simulink model "sample"  (R2018b)
settings: Solver=FixedStepDiscrete  StartTime=0.0  StopTime=10.0  RelTol=1e-3
settings Model: Creator=a_miyazaki  LastModifiedBy=a_miyazaki

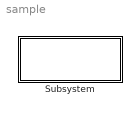
== system sample ==
  Subsystem : Subsystem

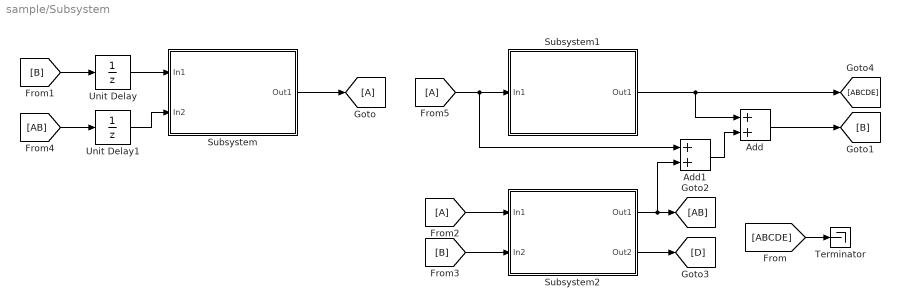
== system sample/Subsystem ==
  Add : Sum
  Add1 : Sum
  Subsystem : Subsystem
  Subsystem1 : Subsystem
  Subsystem2 : Subsystem
  Terminator : Terminator
  Unit Delay : UnitDelay  SampleTime=-1
  Unit Delay1 : UnitDelay  SampleTime=-1
  wires:
  Subsystem2/2(Out2) -> [D]
  [AB] -> Unit Delay1/1
  Add/1 -> [B]
  Unit Delay1/1 -> Subsystem/2(In2)
  Subsystem/1(Out1) -> [A]
  [A] -> Add1/1, Subsystem1/1(In1)
  [B] -> Subsystem2/2(In2)
  Subsystem1/1(Out1) -> [ABCDE], Add/1
  [A] -> Subsystem2/1(In1)
  [B] -> Unit Delay/1
  Subsystem2/1(Out1) -> Add1/2, [AB]
  Unit Delay/1 -> Subsystem/1(In1)
  Add1/1 -> Add/2
  [ABCDE] -> Terminator/1

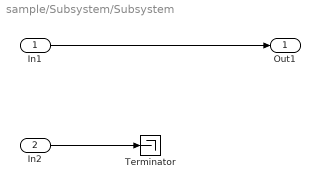
== system sample/Subsystem/Subsystem ==
  In1 : Inport
  In2 : Inport  Port=2
  Terminator : Terminator
  Out1 : Outport
  wires:
  In1/1 -> Out1/1
  In2/1 -> Terminator/1

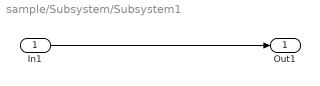
== system sample/Subsystem/Subsystem1 ==
  In1 : Inport
  Out1 : Outport
  wires:
  In1/1 -> Out1/1

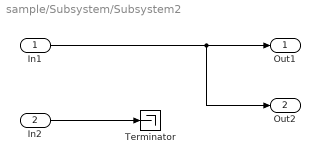
== system sample/Subsystem/Subsystem2 ==
  In1 : Inport
  In2 : Inport  Port=2
  Terminator : Terminator
  Out1 : Outport
  Out2 : Outport  Port=2
  wires:
  In1/1 -> Out2/1, Out1/1
  In2/1 -> Terminator/1
